simulink model "thetapid"  (R2018b)
settings: Solver=VariableStepAuto  StartTime=0.0  StopTime=10.0  RelTol=1e-3  EnableMultiTasking=on
undefined symbols (not defined in the file or in its folder): Kd, Ki, Kp
settings Model: Creator=田振东  LastModifiedBy=12038
settings OptimizationCC: LifeSpan=inf
settings DebuggingCC: SFUnexpectedBacktrackingDiag=warning  SFNoUnconditionalDefaultTransitionDiag=warning
settings SFSimCC: SimUseLocalCustomCode=off
settings RTWCC: RTWUseLocalCustomCode=off
settings CodeAppCC: StateflowObjectComments=on
settings GRTTargetCC: TargetLangStandard=C89/C90 (ANSI)  GeneratePreprocessorConditionals=Disable all
settings ConfigComp: CovMetricSettings=dw  CovHtmlReporting=on  CovSaveCumulativeToWorkspaceVar=on  CovSaveSingleToWorkspaceVar=on  CovExternalEMLEnable=off

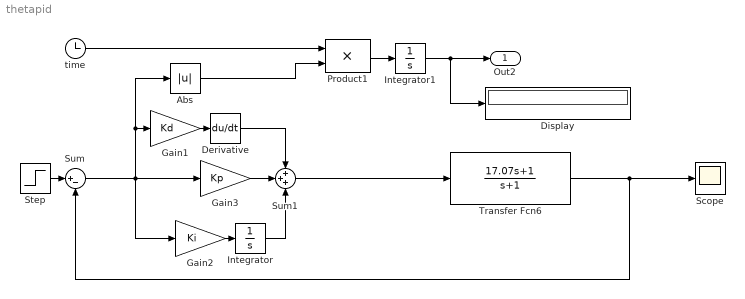
== system thetapid ==
  Abs : Abs  ZeroCross=off  SaturateOnIntegerOverflow=on
  Derivative : Derivative
  Display : Display
  Gain1 : Gain  Gain=Kd
  Gain2 : Gain  Gain=Ki
  Gain3 : Gain  Gain=Kp
  Integrator : Integrator
  Integrator1 : Integrator
  Product1 : Product  SaturateOnIntegerOverflow=on  OutDataTypeStr=Inherit: Same as first input
  Scope : Scope
  Step : Step  Time=0  SampleTime=0
  Sum : Sum  Inputs=|+-  SaturateOnIntegerOverflow=on
  Sum1 : Sum  Inputs=+++  SaturateOnIntegerOverflow=on
  Transfer Fcn6 : TransferFcn  Numerator=[17.07 1]  Denominator=[0 0 0 1 1]
  time : Clock
  Out2 : Outport
  wires:
  Step/1 -> Sum/1
  Sum/1 -> Gain2/1, Gain3/1, Gain1/1, Abs/1
  time/1 -> Product1/1
  Integrator1/1 -> Out2/1, Display/1
  Product1/1 -> Integrator1/1
  Abs/1 -> Product1/2
  Gain3/1 -> Sum1/2
  Integrator/1 -> Sum1/3
  Derivative/1 -> Sum1/1
  Sum1/1 -> Transfer Fcn6/1
  Transfer Fcn6/1 -> Scope/1, Sum/2
  Gain1/1 -> Derivative/1
  Gain2/1 -> Integrator/1
